simulink model "inverted_pendulum"  (R2021a)
settings: Solver=FixedStepAuto  StartTime=0.0  StopTime=20  FixedStep=0.001  MaxStep=0.001  RelTol=1e-3
values from neighbouring files (symbols this model uses):
  d = 0.0    (= 0)    [inverted_pendulum_data.m]
  g = 9.81    [inverted_pendulum_data.m]    (also in pendulumGIF.m; pendulumVideo.m)
  l = 1    [inverted_pendulum_data.m]    (also in pendulumGIF.m = 2; pendulumVideo.m = 2)
  m = 1    [inverted_pendulum_data.m]    (also in pendulumGIF.m; pendulumVideo.m)
  omega_0 = 0.0    (= 0)    [inverted_pendulum_data.m]
  theta_0 = 0.0    (= 0)    [inverted_pendulum_data.m]
libraries: simulink_extras x1
settings Model: Creator=lennartfuhrig  LastModifiedBy=lennartfuhrig

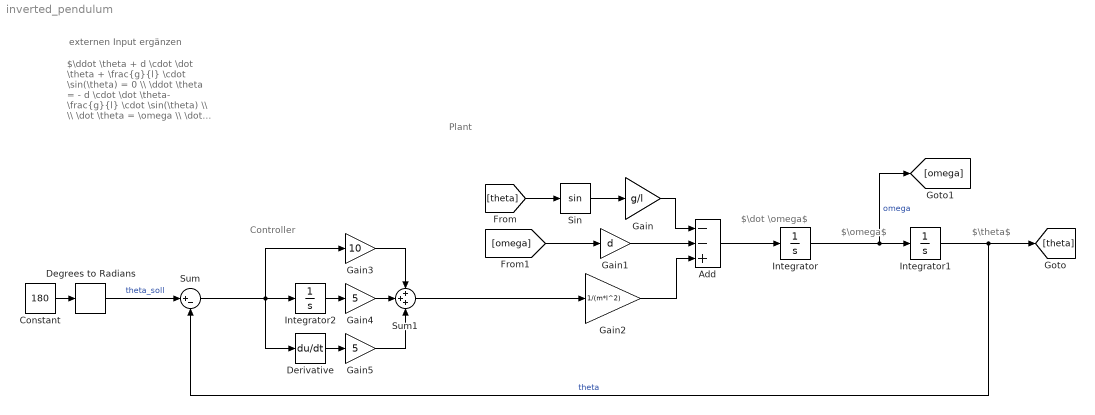
== system inverted_pendulum ==
  note: externen Input ergänzen
  note: Plant
  note: Controller
  note: $\dot \omega$
  note: $\omega$
  note: $\theta$
  note: $\ddot \theta + d \cdot \dot \theta + \frac{g}{l} \cdot \sin(\theta) = 0 \\ \ddot \theta = - d \cdot \dot \theta- \frac{g}{l} \cdot \sin(\theta) \\ \\ \dot \theta = \omega \\ \dot \omega = - d \cdot \omega - \frac{g}{l} \cdot \sin(\theta)$
  Add : Sum  Inputs=--+
  Constant : Constant  Value=180
  Degrees to Radians : simulink_extras/Transformations/Degrees to Radians
  Derivative : Derivative
  Gain : Gain  Gain=g/l
  Gain1 : Gain  Gain=d
  Gain2 : Gain  Gain=1/(m*l^2)
  Gain3 : Gain  Gain=10
  Gain4 : Gain  Gain=5
  Gain5 : Gain  Gain=5
  Integrator : Integrator  InitialCondition=omega_0
  Integrator1 : Integrator  InitialCondition=theta_0
  Integrator2 : Integrator
  Sin : Trigonometry
  Sum : Sum  Inputs=|+-
  Sum1 : Sum  Inputs=+++
  wires:
  Integrator/1 -> Integrator1/1, [omega]  "omega"
  Integrator1/1 -> [theta], Sum/2  "theta"
  Sin/1 -> Gain/1
  [theta] -> Sin/1
  Add/1 -> Integrator/1
  Gain/1 -> Add/1
  Gain1/1 -> Add/2
  [omega] -> Gain1/1
  Gain2/1 -> Add/3
  Constant/1 -> Degrees to Radians/1
  Degrees to Radians/1 -> Sum/1  "theta_soll"
  Gain4/1 -> Sum1/2
  Gain5/1 -> Sum1/3
  Gain3/1 -> Sum1/1
  Integrator2/1 -> Gain4/1
  Derivative/1 -> Gain5/1
  Sum/1 -> Derivative/1, Gain3/1, Integrator2/1
  Sum1/1 -> Gain2/1
